simulink model "IF_Align"  (R2016a)
settings: Solver=VariableStepAuto  StartTime=0.0  StopTime=20*FftSize*Ts  RelTol=1e-3
InitFcn:
  | Ts=3/280e6
  | Br=1/(10*Ts)
  | EbNo=50
  | EbNo2=50
  | FftSize=256
undefined symbols (not defined in the file or in its folder): Offset, Radix
libraries: simulink x3, dspxfrm3 x3, hdlsllib x2, dspsigops x1, commchan3 x1, dspfdesign x1, commdigbbndpm3 x1, commrandsrc3 x1
settings Model: Creator=frank  LastModifiedBy=frank

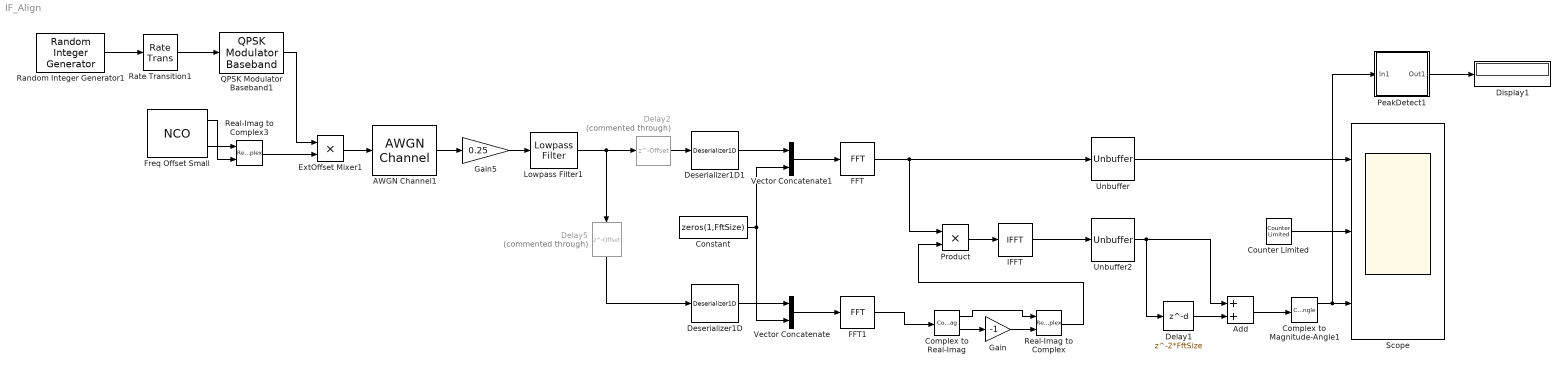
== system IF_Align ==
  " Freq Offset Small" : dspsigops/NCO  AccIncSrc=Specify via dialog  AccInc=floor(10000*Ts*(2^18))  PhaseOffsetSrc=Specify via dialog  PhaseOffset=0  AccumWL=18  HasDither=off  DitherWL=4  PNgeneratorLength=19  HasPhaseQuantizer=off  TableDepth=12  HasOutputPhaseError=off  Formula=Sine and cosine  DataType=double  OutputWL=16  OutputFL=14  CompMethod=Table lookup (no interpolation)  SampleTime=Ts  SamplesPerFrame=1  OutputFrames=off
  AWGN Channel1 : commchan3/AWGN Channel  InputProcessing=Columns as channels (frame based)  seed=67  noiseMode="Signal to noise ratio  (Eb/No)"  EbNodB=EbNo  EsNodB=10  SNRdB=10  bitsPerSym=2  Ps=1  Tsym=1/Br  variance=1
  Add : Sum
  Complex to Magnitude-Angle1 : ComplexToMagnitudeAngle
  Complex to Real-Imag : ComplexToRealImag
  Constant : Constant  Value=zeros(1,FftSize)
  Counter Limited : simulink/Sources/Counter Limited  uplimit=FftSize-1  tsamp=-1
  Delay1 : Delay  DelayLength=2*FftSize
  Delay2 : Delay  Commented=through  DelayLength=Offset
  Delay5 : Delay  Commented=through  DelayLength=Offset
  Deserializer1D : hdlsllib/HDL Operations/Deserializer1D  Ratio=FftSize  IdleCycles=0  InitialCondition=0  startIn=off  validIn=off  validOut=off  inputDataDimensions=-1  inputSampleTime=-1  inputSignalType=auto
  Deserializer1D1 : hdlsllib/HDL Operations/Deserializer1D  Ratio=FftSize  IdleCycles=0  InitialCondition=0  startIn=off  validIn=off  validOut=off  inputDataDimensions=-1  inputSampleTime=-1  inputSignalType=auto
  Display1 : Display
  ExtOffset Mixer1 : Product
  FFT : dspxfrm3/FFT  FFTImplementation=Auto  CompMethod=Table lookup  TableOpt=NEW  TableOptActive=Speed  BitRevOrder=off  Normalize=off  InheritFFTLength=on  FFTLength=256  WrapInput=on  roundingMode=Floor  overflowMode=off  firstCoeffDataTypeStr=Inherit: Same word length as input  firstCoeffLastDataTypeStr=Inherit: Same word length as input  outputMin=[]  outputMax=[]
  FFT1 : dspxfrm3/FFT  FFTImplementation=Auto  CompMethod=Table lookup  TableOpt=NEW  TableOptActive=Speed  BitRevOrder=off  Normalize=off  InheritFFTLength=on  FFTLength=256  WrapInput=on  roundingMode=Floor  overflowMode=off  firstCoeffDataTypeStr=Inherit: Same word length as input  firstCoeffLastDataTypeStr=Inherit: Same word length as input  outputMin=[]  outputMax=[]
  Gain : Gain  Gain=-1
  Gain5 : Gain  Gain=0.25
  IFFT : dspxfrm3/IFFT  FFTImplementation=Radix-2  CompMethod=Table lookup  TableOpt=NEW  TableOptActive=Speed  BitRevOrder=off  cs_in=off  Normalize=on  InheritFFTLength=on  FFTLength=64  WrapInput=on  mode=Complex  outSamplingMode=Sample based  roundingMode=Floor  overflowMode=off  firstCoeffDataTypeStr=Inherit: Same word length as input  firstCoeffLastDataTypeStr=Inherit: Same word length as input  outputMin=[]  outputMax=[]
  Lowpass Filter1 : dspfdesign/Lowpass Filter  FilterType=FIR  DesignForMinimumOrder=on  FilterOrder=50  PassbandFrequency=Br/2  StopbandFrequency=Br*2  PassbandRipple=0.1  StopbandAttenuation=80  InheritSampleRate=off  SampleRate=1/Ts  roundingMode=Floor  coeffsDataTypeStr=fixdt(1,16)  SimulateUsing=Interpreted execution
  PeakDetect1 : Subsystem
  Product : Product
  QPSK Modulator Baseband1 : commdigbbndpm3/QPSK Modulator Baseband  InType=Integer  Enc=Gray  Ph=pi/4  outDtype=double  outWordLen=16  outUDDataType=sfix(16)  outFracLenMode=Best precision  outFracLen=15  outDataTypeStr=double  outLastDataTypeStr=double
  Random Integer Generator1 : commrandsrc3/Random Integer Generator  SetSize=4  SeedSource=Auto  Seed=0  SampleTime=1/Br  SamplesPerFrame=1  OutputDataType=double  SimulateUsing=Code generation
  Rate Transition1 : RateTransition  OutPortSampleTime=Ts
  Real-Imag to Complex : RealImagToComplex
  Real-Imag to Complex3 : RealImagToComplex
  Scope : Scope  NumInputPorts=3
  Unbuffer : Unbuffer  SampleBasedProcessing=Same as frame based
  Unbuffer2 : Unbuffer  SampleBasedProcessing=Same as frame based
  Vector Concatenate : Concatenate
  Vector Concatenate1 : Concatenate
  wires:
  AWGN Channel1/1 -> Gain5/1
  Gain5/1 -> Lowpass Filter1/1
  Random Integer Generator1/1 -> Rate Transition1/1
  Rate Transition1/1 -> QPSK Modulator Baseband1/1
  Lowpass Filter1/1 -> Delay5/1, Delay2/1
  FFT/1 -> Unbuffer/1, Product/1
  Unbuffer/1 -> Scope/1
  Vector Concatenate/1 -> FFT1/1
  Product/1 -> IFFT/1
  IFFT/1 -> Unbuffer2/1
  Vector Concatenate1/1 -> FFT/1
  Delay5/1 -> Deserializer1D/1
  Deserializer1D/1 -> Vector Concatenate/1
  Deserializer1D1/1 -> Vector Concatenate1/1
  Constant/1 -> Vector Concatenate/2, Vector Concatenate1/2
  Unbuffer2/1 -> Add/1, Delay1/1
  Delay1/1 -> Add/2
  " Freq Offset Small"/1 -> Real-Imag to Complex3/2
  " Freq Offset Small"/2 -> Real-Imag to Complex3/1
  Real-Imag to Complex3/1 -> ExtOffset Mixer1/2
  QPSK Modulator Baseband1/1 -> ExtOffset Mixer1/1
  Counter Limited/1 -> Scope/2
  Add/1 -> Complex to Magnitude-Angle1/1
  Complex to Magnitude-Angle1/1 -> PeakDetect1/1(In1), Scope/3
  Gain/1 -> Real-Imag to Complex/2
  Complex to Real-Imag/2 -> Gain/1
  Complex to Real-Imag/1 -> Real-Imag to Complex/1
  FFT1/1 -> Complex to Real-Imag/1
  Real-Imag to Complex/1 -> Product/2
  Delay2/1 -> Deserializer1D1/1
  ExtOffset Mixer1/1 -> AWGN Channel1/1
  PeakDetect1/1(Out1) -> Display1/1

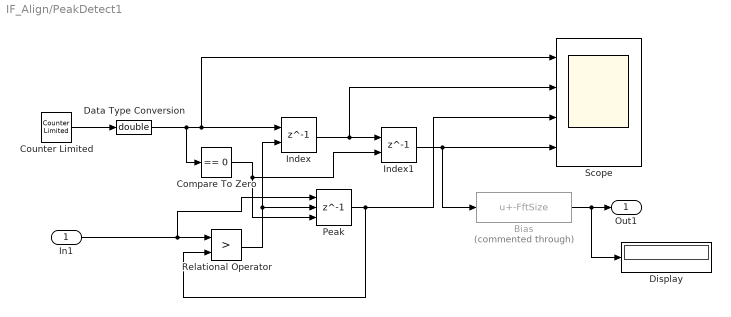
== system IF_Align/PeakDetect1 ==
  In1 : Inport
  Bias : Bias  Commented=through  Bias=-FftSize
  Compare To Zero : simulink/Logic and Bit Operations/Compare To Zero  relop===  OutDataTypeStr=boolean
  Counter Limited : simulink/Sources/Counter Limited  uplimit=FftSize-1  tsamp=-1
  Data Type Conversion : DataTypeConversion  OutDataTypeStr=double
  Display : Display
  Index : Delay  DelayLength=1  ShowEnablePort=on
      settings: InputPortMap=u0,e6
  Index1 : Delay  DelayLength=1  ShowEnablePort=on
      settings: InputPortMap=u0,e6
  Peak : Delay  DelayLength=1  ExternalReset=Rising  ShowEnablePort=on
      settings: InputPortMap=u0,e6,r5
  Relational Operator : RelationalOperator  Operator=>  OutDataTypeStr=boolean
  Scope : Scope  NumInputPorts=4
  Out1 : Outport
  wires:
  Data Type Conversion/1 -> Index/1, Scope/1, Compare To Zero/1
  Bias/1 -> Out1/1, Display/1
  Index1/1 -> Scope/4, Bias/1
  Compare To Zero/1 -> Peak/3, Index1/2
  Relational Operator/1 -> Peak/2, Index/2
  Index/1 -> Index1/1, Scope/2
  Peak/1 -> Relational Operator/2, Scope/3
  In1/1 -> Peak/1, Relational Operator/1
  Counter Limited/1 -> Data Type Conversion/1
